simulink model "Simulink_ZT_P3"  (R2021a)
settings: Solver=FixedStepAuto  StartTime=0.0  StopTime=20  FixedStep=0.0001  RelTol=1e-3
values from neighbouring files (symbols this model uses):
  kT = kTRnf * inv(TRnf)    [Praktikum.m]    (also in ackerSelfmade.m)
  V = -(ZRM.C*(ZRM.A - ZRM.B * kT)^-1 * ZRM.B)^-1    [Praktikum.m]
  wsoll = 0.2    [Praktikum.m]
  x0 = [0 0 0 0]    [Praktikum.m]    (also in Praktikum_1.m = [5 0 0 0])
  z0 = 0    [Praktikum.m]
  zeitverzoegerung = 1    [Praktikum.m]
  ZRM = ZRMGummi    [Praktikum.m]    (also in Praktikum_1.m = ss(A,bv,cT,d); calcZRM.m = ss(A,bv,cT,d))
settings Model: Creator=Origilon  LastModifiedBy=janis
settings SolverCC: AlgebraicLoopSolver=TrustRegion
settings DebuggingCC: SFMachineParentedDataDiag=warning
settings SFSimCC: CustomCodeUndefinedFunction=UseInterfaceOnly

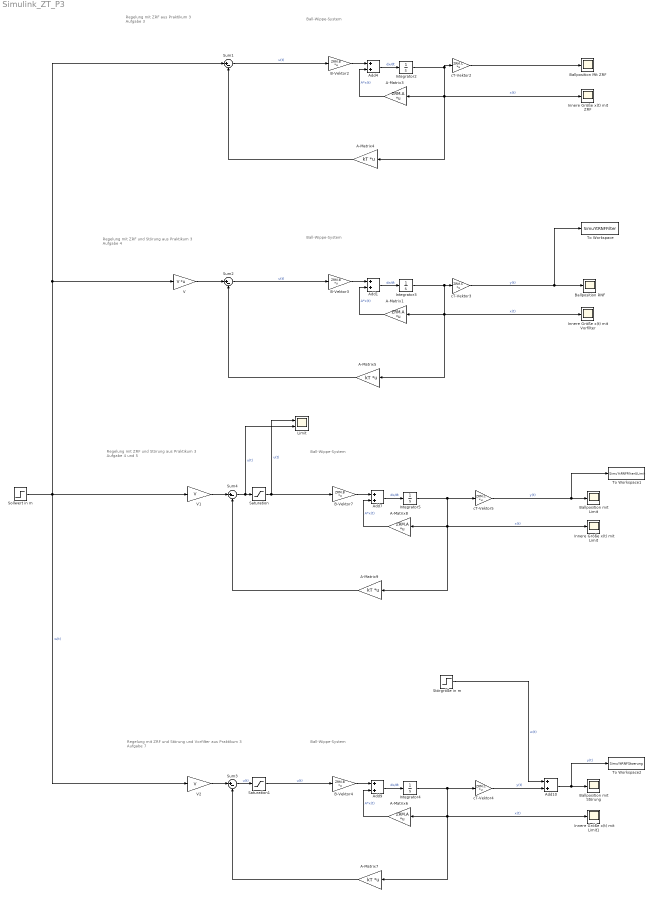
== system Simulink_ZT_P3 ==
  note: Regelung mit ZRF aus Praktikum 3
      |  Aufgabe 3
  note: Ball-Wippe-System
  note: Regelung mit ZRF und Störung aus Praktikum 3
      |  Aufgabe 4
  note: Regelung mit ZRF und Störung und Vorfilter aus Praktikum 3
      | Aufgabe 7
  note: Ball-Wippe-System
  note: Regelung mit ZRF und Störung aus Praktikum 3
      |  Aufgabe 4 und 5
  note: Ball-Wippe-System
  note: Ball-Wippe-System
  A-Matrix{1,3,6,8} (4 alike) : Gain  Gain=ZRM.A  Multiplication=Matrix(K*u) (u vector)
  A-Matrix{4..5,7,9} (4 alike) : Gain  Gain=kT  Multiplication=Matrix(K*u) (u vector)
  Add{1,4,7,9..10} (5 alike) : Sum
  B-Vektor{2..4,7} (4 alike) : Gain  Gain=ZRM.B  Multiplication=Matrix(K*u) (u vector)
  Ballposition Mit ZRF : Scope
  Ballposition RNF : Scope
  Ballposition mit Limit : Scope
  Ballposition mit Störung : Scope
  Innere Größe x(t) mit Limit : Scope
  Innere Größe x(t) mit Limit1 : Scope
  Innere Größe x(t) mit Vorfilter : Scope
  Innere Größe x(t) mit ZRF : Scope
  Integrator{2..5} (4 alike) : Integrator  InitialCondition=x0
  Limit : Scope  NumInputPorts=2
  Saturation : Saturate  UpperLimit=6.45  LowerLimit=-6.45
  Saturation1 : Saturate  UpperLimit=6.45  LowerLimit=-6.45
  Sollwert in m : Step  Time=zeitverzoegerung  After=wsoll  SampleTime=0
  Störgröße in m : Step  Time=10  After=z0  SampleTime=0
  Sum{1..4} (4 alike) : Sum  Inputs=|+-
  To Workspace : ToWorkspace  VariableName=SimuYtRNFFilter  SaveFormat=Timeseries  SampleTime=-1
  To Workspace1 : ToWorkspace  VariableName=SimuYtRNFFilterULimit  SaveFormat=Timeseries  SampleTime=-1
  To Workspace2 : ToWorkspace  VariableName=SimuYtRNFStoerung  SaveFormat=Timeseries  SampleTime=-1
  V : Gain  Gain=V  Multiplication=Matrix(K*u)
  V1 : Gain  Gain=V
  V2 : Gain  Gain=V
  cT-Vektor{2..5} (4 alike) : Gain  Gain=ZRM.C  Multiplication=Matrix(K*u) (u vector)
  wires:
  Add4/1 -> Integrator2/1  "dx/dt"
  cT-Vektor2/1 -> Ballposition Mit ZRF/1
  Sollwert in m/1 -> V2/1, Sum1/1, V/1, V1/1  "w(t)"
  A-Matrix3/1 -> Add4/2  "A*x(t)"
  A-Matrix4/1 -> Sum1/2
  B-Vektor2/1 -> Add4/1
  Sum1/1 -> B-Vektor2/1  "u(t)"
  Integrator2/1 -> cT-Vektor2/1, Innere Größe x(t) mit ZRF/1, A-Matrix4/1, A-Matrix3/1  "x(t)"
  Integrator3/1 -> cT-Vektor3/1, Innere Größe x(t) mit Vorfilter/1, A-Matrix5/1, A-Matrix1/1  "x(t)"
  B-Vektor3/1 -> Add1/1
  A-Matrix1/1 -> Add1/2  "A*x(t)"
  A-Matrix5/1 -> Sum2/2
  Add1/1 -> Integrator3/1  "dx/dt"
  cT-Vektor3/1 -> To Workspace/1, Ballposition RNF/1  "y(t)"
  V/1 -> Sum2/1
  Sum2/1 -> B-Vektor3/1  "u(t)"
  Saturation/1 -> Limit/1, B-Vektor7/1  "u(t)"
  cT-Vektor5/1 -> To Workspace1/1, Ballposition mit Limit/1  "y(t)"
  V1/1 -> Sum4/1
  Add7/1 -> Integrator5/1  "dx/dt"
  B-Vektor7/1 -> Add7/1
  A-Matrix8/1 -> Add7/2  "A*x(t)"
  A-Matrix9/1 -> Sum4/2
  Integrator5/1 -> cT-Vektor5/1, A-Matrix9/1, A-Matrix8/1, Innere Größe x(t) mit Limit/1  "x(t)"
  Sum4/1 -> Limit/2, Saturation/1  "u(t)"
  V2/1 -> Sum3/1
  Add9/1 -> Integrator4/1  "dx/dt"
  Add10/1 -> To Workspace2/1, Ballposition mit Störung/1  "y(t)"
  A-Matrix7/1 -> Sum3/2
  Integrator4/1 -> cT-Vektor4/1, A-Matrix7/1, A-Matrix6/1, Innere Größe x(t) mit Limit1/1  "x(t)"
  B-Vektor4/1 -> Add9/1
  A-Matrix6/1 -> Add9/2  "A*x(t)"
  Sum3/1 -> Saturation1/1  "u(t)"
  Saturation1/1 -> B-Vektor4/1  "u(t)"
  cT-Vektor4/1 -> Add10/2  "y(t)"
  Störgröße in m/1 -> Add10/1  "w(t)"
